simulink model "activity_2"  (R2022a)
settings: Solver=FixedStepAuto  StartTime=0.0  StopTime=5  FixedStep=0.01  RelTol=1e-3
settings Model: Creator=optiplex3060  LastModifiedBy=zhong
settings SolverCC: AlgebraicLoopSolver=TrustRegion
settings DataIOCC: ReturnWorkspaceOutputs=off
settings DebuggingCC: UnconnectedInputMsg=warning  UnconnectedOutputMsg=warning  UnconnectedLineMsg=warning  SFMachineParentedDataDiag=warning  ArithmeticOperatorsInVariantConditions=warning
settings SFSimCC: CustomCodeUndefinedFunction=UseInterfaceOnly

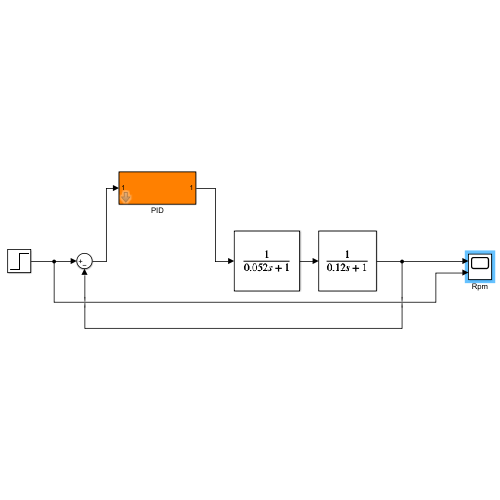
[thumbnail: Simulink's stored preview of the top-level diagram]
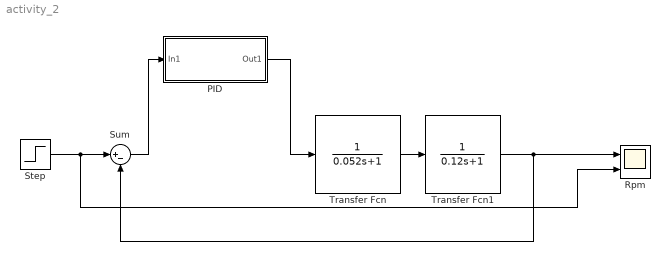
== system activity_2 ==
  PID : Subsystem  mask{Kp=1, Ki=0, Kd=0}
      mask DialogControl ParameterGroupVar Prompt: 参数
  "Rpm " : Scope  NumInputPorts=2
  Step : Step  After=2000  SampleTime=0
  Sum : Sum  Inputs=|+-
  Transfer Fcn : TransferFcn  Denominator=[0.052 1]
  Transfer Fcn1 : TransferFcn  Denominator=[0.12 1]
  wires:
  Step/1 -> "Rpm "/2, Sum/1
  Transfer Fcn/1 -> Transfer Fcn1/1
  Transfer Fcn1/1 -> Sum/2, "Rpm "/1
  Sum/1 -> PID/1(In1)
  PID/1(Out1) -> Transfer Fcn/1

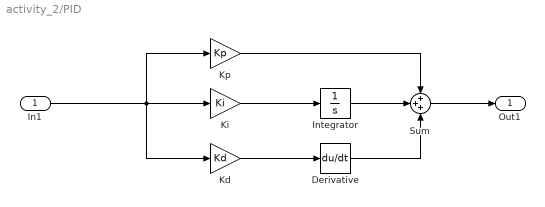
== system activity_2/PID ==
  In1 : Inport
  Derivative : Derivative
  Integrator : Integrator
  Kd : Gain  Gain=Kd
  Ki : Gain  Gain=Ki
  "Kp " : Gain  Gain=Kp
  Sum : Sum  Inputs=+++
  Out1 : Outport  VectorParamsAs1DForOutWhenUnconnected=off
  wires:
  In1/1 -> Kd/1, "Kp "/1, Ki/1
  Kd/1 -> Derivative/1
  Ki/1 -> Integrator/1
  "Kp "/1 -> Sum/1
  Integrator/1 -> Sum/2
  Derivative/1 -> Sum/3
  Sum/1 -> Out1/1
